simulink model "SafetySOMANET"  (R2016b)
settings: Solver=VariableStepAuto  StartTime=0.0  StopTime=10.0  RelTol=1e-3
settings Model: DataDictionary=ModelDictionary.sldd  Creator=Nathan  LastModifiedBy=Nathan

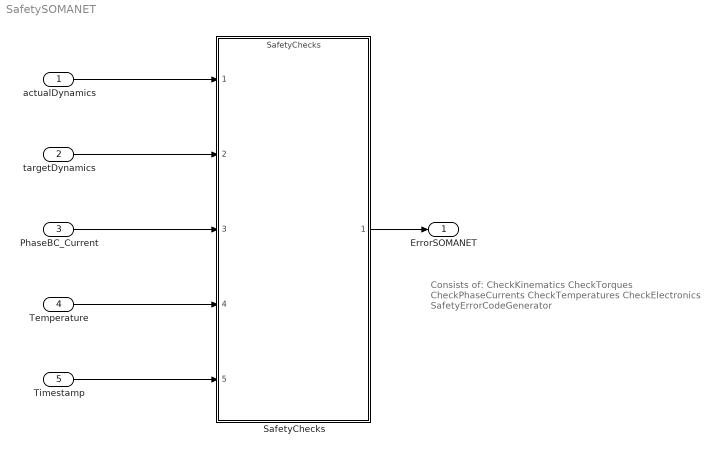
== system SafetySOMANET ==
  note: Consists of:
      | CheckKinematics
      | CheckTorques
      | CheckPhaseCurrents
      | CheckTemperatures
      | CheckElectronics
      | SafetyErrorCodeGenerator
  actualDynamics : Inport  OutDataTypeStr=Bus: actualDynamics  BusOutputAsStruct=on
  targetDynamics : Inport  Port=2  OutDataTypeStr=Bus: targetDynamics  BusOutputAsStruct=on
  PhaseBC_Current : Inport  Port=3  OutDataTypeStr=Bus: PhaseBC_Current  BusOutputAsStruct=on
  Temperature : Inport  Port=4  BusOutputAsStruct=on
  Timestamp : Inport  Port=5  BusOutputAsStruct=on
  SafetyChecks : ModelReference  ModelNameDialog=SafetyChecks.slx  SimulationMode=Normal  ModelReferenceVersion=1.15
  ErrorSOMANET : Outport
  wires:
  SafetyChecks/1 -> ErrorSOMANET/1
  actualDynamics/1 -> SafetyChecks/1
  targetDynamics/1 -> SafetyChecks/2
  PhaseBC_Current/1 -> SafetyChecks/3
  Temperature/1 -> SafetyChecks/4
  Timestamp/1 -> SafetyChecks/5
